simulink model "DC_AC"  (R2023a)
settings: Solver=VariableStepAuto  StartTime=0.0  StopTime=1.5  MaxStep=1e-4  RelTol=1e-3
libraries: spsMosfetLib x32, spsSeriesRLCBranchLib x29, simulink x25, spsCurrentMeasurementLib x11, spsVoltageMeasurementLib x9, spsDCVoltageSourceLib x8, spsIdealSwitchLib x5, spsDiodeLib x1, spspowerguiLib x1
(part 1 of 2)
settings Model: Creator=TangZhenYu  LastModifiedBy=TangZhenYu

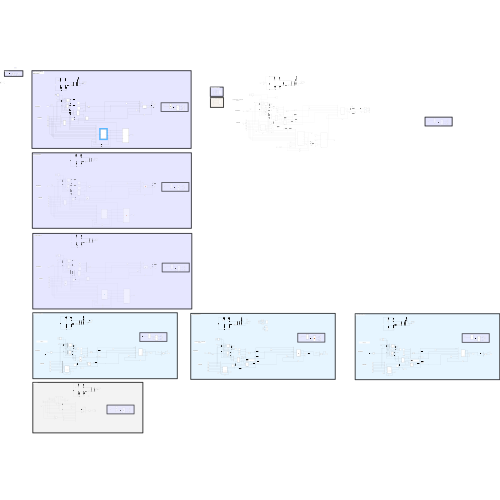
[thumbnail: Simulink's stored preview of the top-level diagram]
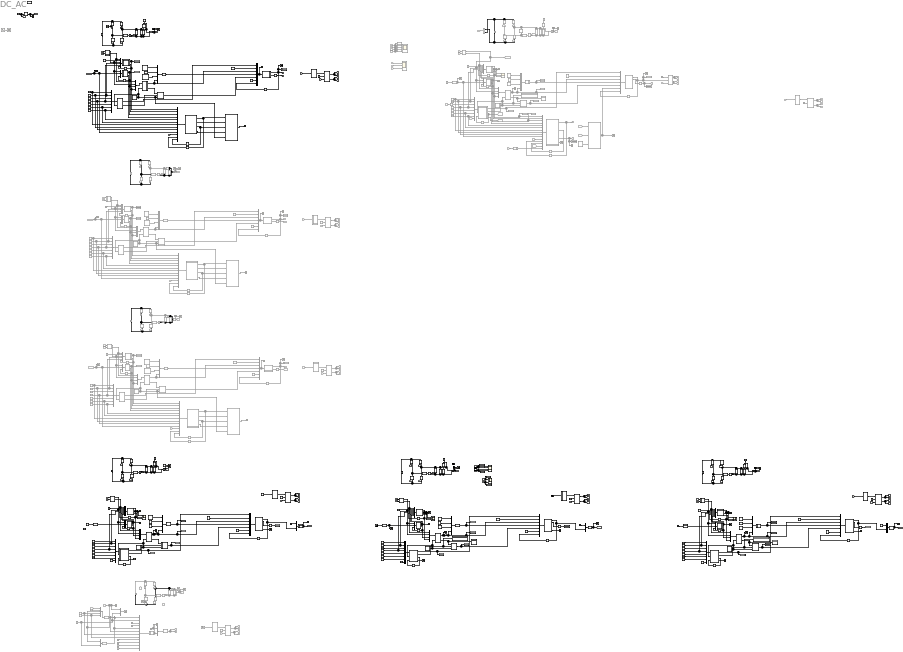
== system DC_AC ==
  note: 固定扰动下的电压跟踪效果
  note: 产生期望值
  note: 不同参数矩阵C下电压跟踪的状态
  note: C矩阵参数设置[1000,1]
  note: 最终驱动
  note: 电路参数
  note: 期望值修改
  note: 期望值修改
  note: 最终驱动
  note: 电路参数
  note: C矩阵参数设置[500,1],500的效果最好
  note: C矩阵参数设置[1500,1]
  note: 电路参数
  note: 最终驱动
  note: 期望值修改
  note: 注意代数环要延时一个机器周期的时间长度
  note: 期望值修改
  note: 电路参数
  note: 不考虑外部扰动的滑膜控制
  note: 最终驱动
  note: 传统的滑膜控制
  note: 最终驱动
  note: 注意代数环要延时一个机器周期的时间长度
  note: 电路参数
  note: 期望值修改
  note: 最终驱动
  note: 注意代数环要延时一个机器周期的时间长度
  note: 期望值修改
  note: 电路参数
  note: 不考虑外部扰动的滑膜控制
  note: 最终驱动
  note: 不考虑外部扰动的滑膜控制
  note: 期望值修改
  note: 最终驱动
  note: 注意代数环要延时一个机器周期的时间长度
  note: 电路参数
  (CΓ)'_Calculation : MATLAB Function  TreatAsAtomicUnit=on
  (CΓ)'_Calculation1 : MATLAB Function  Commented=on  TreatAsAtomicUnit=on
  (CΓ)'_Calculation2 : MATLAB Function  Commented=on  TreatAsAtomicUnit=on
  (CΓ)'_Calculation3 : MATLAB Function  TreatAsAtomicUnit=on
  (CΓ)'_Calculation4 : MATLAB Function  Commented=on  TreatAsAtomicUnit=on
  (CΓ)'_Calculation5 : MATLAB Function  TreatAsAtomicUnit=on
  (CΓ)'_Calculation6 : MATLAB Function  TreatAsAtomicUnit=on
  C : Constant  Commented=on  Value=1e-5
  C(电容值) : Constant  Value=1e-3
  C(电容值)1 : Constant  Commented=on  Value=1e-3
  C(电容值)2 : Constant  Commented=on  Value=1e-3
  C(电容值)3 : Constant  Value=0.0003
  C(电容值)4 : Constant  Commented=on  Value=0.0003
  C(电容值)5 : Constant  Value=0.0003
  C(电容值)6 : Constant  Value=0.0003
  C1 : Constant  Commented=on  Value=100
  C_Gamma_Inv1 : Display
  C_Gamma_Inv2 : Display
  C_Gamma_Inv3 : Display
  C_Gamma_Inv4 : Display  Commented=on
  Constant : Constant  Commented=on  Value=30
  Constant{1..5} (5 alike) : Constant  Commented=on  Value=0
  Current Measurement{1..3,6..7,12..13} (7 alike) : spsCurrentMeasurementLib/Current Measurement  Commented=on  PhasorSimulation=off  OutputType=Complex  PSBequivalent=0
  Current Measurement{4..5,8..9} (4 alike) : spsCurrentMeasurementLib/Current Measurement  PhasorSimulation=off  OutputType=Complex  PSBequivalent=0
  Cϕx1 : Display
  Cϕx2 : Display
  Cϕx3 : Display
  Cϕx4 : Display  Commented=on
  Cϕx_Calculation : MATLAB Function  TreatAsAtomicUnit=on
  Cϕx_Calculation1 : MATLAB Function  Commented=on  TreatAsAtomicUnit=on
  Cϕx_Calculation2 : MATLAB Function  Commented=on  TreatAsAtomicUnit=on
  Cϕx_Calculation3 : MATLAB Function  TreatAsAtomicUnit=on
  Cϕx_Calculation4 : MATLAB Function  Commented=on  TreatAsAtomicUnit=on
  Cϕx_Calculation5 : MATLAB Function  TreatAsAtomicUnit=on
  Cϕx_Calculation6 : MATLAB Function  TreatAsAtomicUnit=on
  DC Voltage Source1 : spsDCVoltageSourceLib/DC Voltage Source  Commented=on  Amplitude=80  Measurements=None
  DC Voltage Source2 : spsDCVoltageSourceLib/DC Voltage Source  Amplitude=80  Measurements=None
  DC Voltage Source3 : spsDCVoltageSourceLib/DC Voltage Source  Commented=on  Amplitude=80  Measurements=None
  DC Voltage Source4 : spsDCVoltageSourceLib/DC Voltage Source  Amplitude=80  Measurements=None
  DC Voltage Source5 : spsDCVoltageSourceLib/DC Voltage Source  Amplitude=85  Measurements=None
  DC Voltage Source6 : spsDCVoltageSourceLib/DC Voltage Source  Amplitude=85  Measurements=None
  DC Voltage Source7 : spsDCVoltageSourceLib/DC Voltage Source  Commented=on  Amplitude=50  Measurements=None
  DC Voltage Source9 : spsDCVoltageSourceLib/DC Voltage Source  Commented=on  Amplitude=80  Measurements=None
  Diode2 : spsDiodeLib/Diode  Commented=on  Ron=0.001  Lon=0  Vf=0.8  IC=0  UseSnubber=0  Rs=500  Cs=250e-9  Measurements=off
  Distrubance_Calculation : MATLAB Function  TreatAsAtomicUnit=on
  Distrubance_Calculation1 : MATLAB Function  TreatAsAtomicUnit=on
  Distrubance_Calculation2 : MATLAB Function  Commented=on  TreatAsAtomicUnit=on
  Distrubance_Calculation3 : MATLAB Function  Commented=on  TreatAsAtomicUnit=on
  Distrubance_Calculation4 : MATLAB Function  Commented=on  TreatAsAtomicUnit=on
  Distrubance_Calculation5 : MATLAB Function  Commented=on  TreatAsAtomicUnit=on
  Distrubance_Calculation6 : MATLAB Function  Commented=on  TreatAsAtomicUnit=on
  Distrubance_Calculation7 : MATLAB Function  Commented=on  TreatAsAtomicUnit=on
  E : Constant  Commented=on  Value=40
  E(实际的值){,3,5..6} (4 alike) : Constant  Value=70
  E(实际的值)1 : Constant  Commented=on  Value=80
  E(实际的值)2 : Constant  Commented=on  Value=80
  E(实际的值)4 : Constant  Commented=on  Value=70
  E_0(理论值){,3,5..6} (4 alike) : Constant  Value=70
  E_0(理论值)1 : Constant  Commented=on  Value=80
  E_0(理论值)2 : Constant  Commented=on  Value=80
  E_0(理论值)4 : Constant  Commented=on  Value=70
  From11 : From  Commented=on  GotoTag=Q1_2
  From14 : From  Commented=on  GotoTag=Q2_2
  From15 : From  Commented=on  GotoTag=u_k_2
  From16 : From  Commented=on  GotoTag=Q1_3
  From17 : From  Commented=on  GotoTag=Q2_3
  From18 : From  Commented=on  GotoTag=u_k_3
  From19 : From  Commented=on  GotoTag=Q3_3
  From20 : From  Commented=on  GotoTag=Q4_3
  From21 : From  Commented=on  GotoTag=u_k_1_3
  From22 : From  Commented=on  GotoTag=v_o_3
  From23 : From  Commented=on  GotoTag=i_l_3
  From24 : From  Commented=on  GotoTag=v_o
  From25 : From  Commented=on  GotoTag=v_o_2
  From26 : From  Commented=on  GotoTag=v_o_3
  From34 : From  Commented=on  GotoTag=i_l_5
  From35 : From  Commented=on  GotoTag=u_k_5
  From36 : From  Commented=on  GotoTag=v_o_5
  From38 : From  Commented=on  GotoTag=expect_value
  From39 : From  Commented=on  GotoTag=Q1_5
  From40 : From  Commented=on  GotoTag=Q2_5
  From41 : From  Commented=on  GotoTag=Q3_5
  From42 : From  Commented=on  GotoTag=Q4_5
  From43 : From  Commented=on  GotoTag=expect_value
  From{45..47,63,79} (5 alike) : From  Commented=on  GotoTag=expect
  From48 : From  Commented=on  GotoTag=v_o
  From49 : From  Commented=on  GotoTag=v_o_4
  From5 : From  Commented=on  GotoTag=Q3_2
  From50 : From  Commented=on  GotoTag=v_o_3
  From53 : From  Commented=on  GotoTag=i_l_6
  From54 : From  Commented=on  GotoTag=V_Output_6
  From55 : From  Commented=on  GotoTag=V_Input_6
  From56 : From  Commented=on  GotoTag=d1_6
  From57 : From  Commented=on  GotoTag=D_Disturb_k_1_6
  From58 : From  Commented=on  GotoTag=D_Disturb_k_2_6
  From59 : From  Commented=on  GotoTag=u_k_1_6
  From6 : From  Commented=on  GotoTag=Q4_2
  From64 : From  Commented=on  GotoTag=v_o_6
  From7 : From  Commented=on  GotoTag=u_k_1_2
  From73 : From  Commented=on  GotoTag=Q3_6
  From74 : From  Commented=on  GotoTag=Q4_6
  From75 : From  Commented=on  GotoTag=Q1_6
  From76 : From  Commented=on  GotoTag=Q2_6
  From8 : From  Commented=on  GotoTag=v_o_2
  From9 : From  Commented=on  GotoTag=i_l_2
  Goto : Goto  Commented=on  GotoTag=Q1_6
  Goto10 : Goto  Commented=on  GotoTag=i_l_2
  Goto11 : Goto  Commented=on  GotoTag=Q4_2
  Goto12 : Goto  Commented=on  GotoTag=Q1_2
  Goto15 : Goto  Commented=on  GotoTag=u_k_1_2
  Goto16 : Goto  Commented=on  GotoTag=u_k_2
  Goto17 : Goto  Commented=on  GotoTag=i_l_3
  Goto18 : Goto  Commented=on  GotoTag=Q4_3
  Goto19 : Goto  Commented=on  GotoTag=Q1_3
  Goto20 : Goto  Commented=on  GotoTag=u_k_1_3
  Goto21 : Goto  Commented=on  GotoTag=u_k_3
  Goto22 : Goto  Commented=on  GotoTag=v_o_3
  Goto23 : Goto  Commented=on  GotoTag=Q2_3
  Goto24 : Goto  Commented=on  GotoTag=Q3_3
  Goto3 : Goto  Commented=on  GotoTag=v_o_2
  Goto33 : Goto  Commented=on  GotoTag=Q4_5
  Goto34 : Goto  Commented=on  GotoTag=Q1_5
  Goto35 : Goto  Commented=on  GotoTag=i_l_5
  Goto36 : Goto  Commented=on  GotoTag=v_o_5
  Goto37 : Goto  Commented=on  GotoTag=Q2_5
  Goto38 : Goto  Commented=on  GotoTag=Q3_5
  Goto40 : Goto  Commented=on  GotoTag=Q4_5
  Goto41 : Goto  Commented=on  GotoTag=Q1_5
  Goto42 : Goto  Commented=on  GotoTag=u_k_1_6
  Goto44 : Goto  Commented=on  GotoTag=V_Output_6
  Goto45 : Goto  Commented=on  GotoTag=R_6
  Goto46 : Goto  Commented=on  GotoTag=V_Input_6
  Goto47 : Goto  Commented=on  GotoTag=d1_6
  Goto48 : Goto  Commented=on  GotoTag=D_Disturb_k_1_6
  Goto49 : Goto  Commented=on  GotoTag=D_Disturb_k_2_6
  Goto5 : Goto  Commented=on  GotoTag=Q2_2
  Goto50 : Goto  Commented=on  GotoTag=v_o_6
  Goto51 : Goto  Commented=on  GotoTag=i_l_6
  Goto52 : Goto  Commented=on  GotoTag=Q4_6
  Goto57 : Goto  Commented=on  GotoTag=Q2_6
  Goto58 : Goto  Commented=on  GotoTag=Q3_6
  Goto61 : Goto  Commented=on  GotoTag=Q4_6
  Goto62 : Goto  Commented=on  GotoTag=Q1_6
  Goto63 : Goto  Commented=on  GotoTag=Q2_6
  Goto64 : Goto  Commented=on  GotoTag=Q3_6
  Goto9 : Goto  Commented=on  GotoTag=Q3_2
  Ideal Switch{,1,3..4} (4 alike) : spsIdealSwitchLib/Ideal Switch  Ron=0.5  Lon=0  IC=0  Rs=1e5  Cs=inf  Measurements=off
  Ideal Switch2 : spsIdealSwitchLib/Ideal Switch  Commented=on  Ron=0.5  Lon=0  IC=0  Rs=1e5  Cs=inf  Measurements=off
  L : Constant  Commented=on  Value=0.05
  L(电感值){,3,5..6} (4 alike) : Constant  Value=0.00365
  L(电感值)1 : Constant  Commented=on  Value=5e-3
  L(电感值)2 : Constant  Commented=on  Value=5e-3
  L(电感值)4 : Constant  Commented=on  Value=0.00365
  MATLAB Function : MATLAB Function  TreatAsAtomicUnit=on
  MATLAB Function1 : MATLAB Function  TreatAsAtomicUnit=on
  MATLAB Function10 : MATLAB Function  Commented=on  TreatAsAtomicUnit=on
  MATLAB Function11 : MATLAB Function  Commented=on  TreatAsAtomicUnit=on
  MATLAB Function12 : MATLAB Function  TreatAsAtomicUnit=on
  MATLAB Function13 : MATLAB Function  TreatAsAtomicUnit=on
  MATLAB Function14 : MATLAB Function  TreatAsAtomicUnit=on
  MATLAB Function15 : MATLAB Function  TreatAsAtomicUnit=on
  MATLAB Function16 : MATLAB Function  TreatAsAtomicUnit=on
  MATLAB Function17 : MATLAB Function  TreatAsAtomicUnit=on
  MATLAB Function18 : MATLAB Function  Commented=on  TreatAsAtomicUnit=on
  MATLAB Function19 : MATLAB Function  Commented=on  TreatAsAtomicUnit=on
  MATLAB Function2 : MATLAB Function  Commented=on  TreatAsAtomicUnit=on
  MATLAB Function20 : MATLAB Function  TreatAsAtomicUnit=on
  MATLAB Function21 : MATLAB Function  Commented=on  TreatAsAtomicUnit=on
  MATLAB Function22 : MATLAB Function  TreatAsAtomicUnit=on
  MATLAB Function23 : MATLAB Function  TreatAsAtomicUnit=on
  MATLAB Function24 : MATLAB Function  TreatAsAtomicUnit=on
  MATLAB Function25 : MATLAB Function  Commented=on  TreatAsAtomicUnit=on
  MATLAB Function26 : MATLAB Function  Commented=on  TreatAsAtomicUnit=on
  MATLAB Function27 : MATLAB Function  Commented=on  TreatAsAtomicUnit=on
  MATLAB Function28 : MATLAB Function  Commented=on  TreatAsAtomicUnit=on
  MATLAB Function29 : MATLAB Function  TreatAsAtomicUnit=on
  MATLAB Function3 : MATLAB Function  Commented=on  TreatAsAtomicUnit=on
  MATLAB Function30 : MATLAB Function  TreatAsAtomicUnit=on
  MATLAB Function31 : MATLAB Function  TreatAsAtomicUnit=on
  MATLAB Function32 : MATLAB Function  TreatAsAtomicUnit=on
  MATLAB Function33 : MATLAB Function  TreatAsAtomicUnit=on
  MATLAB Function4 : MATLAB Function  TreatAsAtomicUnit=on
  MATLAB Function5 : MATLAB Function  TreatAsAtomicUnit=on
  MATLAB Function6 : MATLAB Function  Commented=on  TreatAsAtomicUnit=on
  MATLAB Function7 : MATLAB Function  Commented=on  TreatAsAtomicUnit=on
  MATLAB Function8 : MATLAB Function  Commented=on  TreatAsAtomicUnit=on
  MATLAB Function9 : MATLAB Function  Commented=on  TreatAsAtomicUnit=on
  Mosfet{1,6..12,22..25,27..30} (16 alike) : spsMosfetLib/Mosfet  Commented=on  Ron=0.1  Lon=0  Rd=0.01  Vfd=0  IC=0  Rs=1e5  Cs=inf  Measurements=off
  Mosfet{2..5,13..21,26,31..32} (16 alike) : spsMosfetLib/Mosfet  Ron=0.1  Lon=0  Rd=0.01  Vfd=0  IC=0  Rs=1e5  Cs=inf  Measurements=off
  Mux : Mux  Inputs=7
  Mux{1,5,23,27,42,46,49,53} (8 alike) : Mux
  Mux10 : Mux  Commented=on  Inputs=[1 1 1]
  Mux11 : Mux  Commented=on  Inputs=[1 1 1 1 1 1 1 1 1 1 1 1 1]
  Mux{8,12,16,19,34,38} (6 alike) : Mux  Commented=on
  Mux13 : Mux  Commented=on  Inputs=[1 1 1 1 1 1 1]
  Mux14 : Mux  Commented=on  Inputs=[1 1 1]
  Mux15 : Mux  Commented=on  Inputs=[1 1 1 1 1 1 1 1 1 1 1 1 1]
  Mux17 : Mux  Commented=on  Inputs=[1 1 1 1 1 1 1]
  Mux18 : Mux  Commented=on  Inputs=7
  Mux2 : Mux  Inputs=[1 1 1 1 1 1]
  Mux20 : Mux  Commented=on  Inputs=[1 1 1 1 1 1]
  Mux21 : Mux  Inputs=[1 1 1 1 1 1 1 1]
  Mux{3,22,41,48} (4 alike) : Mux  Inputs=[1 1 1]
  Mux{6,24,43,50} (4 alike) : Mux  Inputs=[1 1 1 1 1 1 1]
  Mux25 : Mux  Inputs=[1 1]
  Mux26 : Mux  Inputs=8
  Mux28 : Mux  Commented=on  Inputs=2
  Mux29 : Mux  Commented=on  Inputs=5
  Mux30 : Mux  Commented=on  Inputs=2
  Mux31 : Mux  Commented=on  Inputs=12
  Mux32 : Mux  Commented=on  Inputs=[1 1]
  Mux33 : Mux  Commented=on  Inputs=8
  Mux35 : Mux  Commented=on  Inputs=[1 1 1 1 1 1 1 1]
  Mux36 : Mux  Commented=on  Inputs=[1 1 1]
  Mux37 : Mux  Commented=on  Inputs=[1 1 1 1 1 1 1 1 1 1 1 1 1 1 1]
  Mux39 : Mux  Commented=on  Inputs=[1 1 1 1 1 1 1]
  Mux4 : Mux  Inputs=[1 1 1 1 1 1 1 1 1 1 1 1 1]
  Mux40 : Mux  Inputs=[1 1 1 1 1 1 1 1]
  Mux44 : Mux  Inputs=[1 1]
  Mux45 : Mux  Inputs=8
  Mux47 : Mux  Inputs=[1 1 1 1 1 1 1 1]
  Mux51 : Mux  Inputs=[1 1]
  Mux52 : Mux  Inputs=8
  Mux7 : Mux  Commented=on  Inputs=7
  Mux9 : Mux  Commented=on  Inputs=[1 1 1 1 1 1]
  Phi2 : Display  Commented=on
  Phi3 : Display
  Phi4 : Display
  R(实际值)1 : From  Commented=on  GotoTag=R_6
  R(实际的值) : Constant  Value=50
  R(实际的值)1 : Constant  Commented=on  Value=50
  R(实际的值)2 : Constant  Commented=on  Value=50
  R_0 : Constant  Commented=on  Value=60
  R_0(实际值)1 : Constant  Value=50
  R_0(实际值)2 : Constant  Commented=on  Value=50
  R_0(实际值)3 : Constant  Value=50
  R_0(实际值)4 : Constant  Value=50
  R_0(理论值) : Constant  Value=42
  R_0(理论值)1 : Constant  Commented=on  Value=50
  R_0(理论值)2 : Constant  Commented=on  Value=50
  R_0(理论值)3 : Constant  Value=50
  R_0(理论值)4 : Constant  Commented=on  Value=50
  R_0(理论值)5 : Constant  Value=50
  R_0(理论值)6 : Constant  Value=50
  Real_R_Value1 : Display  Commented=on
  Repeating Sequence Stair{,2..3,8} (4 alike) : simulink/Sources/Repeating Sequence Stair  OutValues=[0 1].'  tsamp=0.05  OutMin=[]  OutMax=[]  OutDataTypeStr=double  OutputDataTypeScalingMode=double  OutDataType=fixdt(0,8)  ConRadixGroup=Best Precision: Vector-wise  OutScaling=2^-12
  Repeating Sequence Stair1 : simulink/Sources/Repeating Sequence Stair  OutValues=[-40 40].'  tsamp=0.1  OutMin=[]  OutMax=[]  OutDataTypeStr=double  OutputDataTypeScalingMode=double  OutDataType=fixdt(0,8)  ConRadixGroup=Best Precision: Vector-wise  OutScaling=2^-12
  Repeating Sequence Stair10 : simulink/Sources/Repeating Sequence Stair  OutValues=[40.2 -40.2].'  tsamp=0.1  OutMin=[]  OutMax=[]  OutDataTypeStr=double  OutputDataTypeScalingMode=double  OutDataType=fixdt(0,8)  ConRadixGroup=Best Precision: Vector-wise  OutScaling=2^-12
  Repeating Sequence Stair11 : simulink/Sources/Repeating Sequence Stair  OutValues=[40.2 -40.2].'  tsamp=0.5  OutMin=[]  OutMax=[]  OutDataTypeStr=double  OutputDataTypeScalingMode=double  OutDataType=fixdt(0,8)  ConRadixGroup=Best Precision: Vector-wise  OutScaling=2^-12
  Repeating Sequence Stair4 : simulink/Sources/Repeating Sequence Stair  Commented=on  OutValues=[0 1].'  tsamp=0.05  OutMin=[]  OutMax=[]  OutDataTypeStr=double  OutputDataTypeScalingMode=double  OutDataType=fixdt(0,8)  ConRadixGroup=Best Precision: Vector-wise  OutScaling=2^-12
  Repeating Sequence Stair5 : simulink/Sources/Repeating Sequence Stair  OutValues=[40.2 -40.2].'  tsamp=0.5  OutMin=[]  OutMax=[]  OutDataTypeStr=double  OutputDataTypeScalingMode=double  OutDataType=fixdt(0,8)  ConRadixGroup=Best Precision: Vector-wise  OutScaling=2^-12
  Repeating Sequence Stair6 : simulink/Sources/Repeating Sequence Stair  OutValues=[40.2 -40.2].'  tsamp=0.5  OutMin=[]  OutMax=[]  OutDataTypeStr=double  OutputDataTypeScalingMode=double  OutDataType=fixdt(0,8)  ConRadixGroup=Best Precision: Vector-wise  OutScaling=2^-12
  Repeating Sequence Stair7 : simulink/Sources/Repeating Sequence Stair  Commented=on  OutValues=[40 -40].'  tsamp=0.1  OutMin=[]  OutMax=[]  OutDataTypeStr=double  OutputDataTypeScalingMode=double  OutDataType=fixdt(0,8)  ConRadixGroup=Best Precision: Vector-wise  OutScaling=2^-12
  Repeating Sequence Stair9 : simulink/Sources/Repeating Sequence Stair  OutValues=[-42 42].'  tsamp=0.1  OutMin=[]  OutMax=[]  OutDataTypeStr=double  OutputDataTypeScalingMode=double  OutDataType=fixdt(0,8)  ConRadixGroup=Best Precision: Vector-wise  OutScaling=2^-12
  Repeating Sequence1 : simulink/Sources/Repeating Sequence  Commented=on  rep_seq_t=[0 0.5/1000 1/1000]  rep_seq_y=[0 1 0]
  Repeating Sequence{2,5,10,12} (4 alike) : simulink/Sources/Repeating Sequence  rep_seq_t=[0 0.5/1000 1/1000]  rep_seq_y=[0 1 0]
  Repeating Sequence11 : simulink/Sources/Repeating Sequence  Commented=on  rep_seq_t=[0 0.5/1000 1/1000]  rep_seq_y=[0 1 0]
  Repeating Sequence13 : simulink/Sources/Repeating Sequence  rep_seq_t=[0 5e-4 10e-4]  rep_seq_y=[0 1.5 0]
  Repeating Sequence3 : simulink/Sources/Repeating Sequence  Commented=on  rep_seq_t=[0 0.5/1000 1/1000]  rep_seq_y=[0 1 0]
  Repeating Sequence4 : simulink/Sources/Repeating Sequence  rep_seq_t=[0 5e-4 10e-4]  rep_seq_y=[0 1.5 0]
  Repeating Sequence6 : simulink/Sources/Repeating Sequence  Commented=on  rep_seq_t=[0 5e-4 10e-4]  rep_seq_y=[0 1 0]
  Repeating Sequence7 : simulink/Sources/Repeating Sequence  Commented=on  rep_seq_t=[0 0.5/1000 1/1000]  rep_seq_y=[0 15 0]
  Repeating Sequence8 : simulink/Sources/Repeating Sequence  Commented=on  rep_seq_t=[0 5e-4 10e-4]  rep_seq_y=[0 1.5 0]
  Repeating Sequence9 : simulink/Sources/Repeating Sequence  rep_seq_t=[0 5e-4 10e-4]  rep_seq_y=[0 1.5 0]
  Scope{,17..18,50,59} (5 alike) : Scope  NumInputPorts=2
  Scope{1,10,30..31,38} (5 alike) : Scope  Commented=on  NumInputPorts=2
  Scope{6..9,11..14,16,21..22,33..34,39,41..44,49,61} (20 alike) : Scope  Commented=on
  Scope15 : Scope  Commented=on  NumInputPorts=4
  Scope{2..5,19,23..29,37,40,45..47,51,53..58,60} (25 alike) : Scope
  Scope20 : Scope  NumInputPorts=3
  Scope32 : Scope  Commented=on  NumInputPorts=3
  Scope35 : Scope  Commented=on  NumInputPorts=3
  Scope36 : Scope  NumInputPorts=3
  Scope48 : Scope  NumInputPorts=4
  Scope52 : Scope  NumInputPorts=3
  Series RLC Branch1 : spsSeriesRLCBranchLib/Series RLC Branch  Commented=on  LConnTagsString=__new0  RConnTagsString=__new0  BranchType=L  Resistance=1  Inductance=5e-3  SetiL0=off  InitialCurrent=0  Capacitance=1e-6  Setx0=off  InitialVoltage=0  Measurements=None
  Series RLC Branch10 : spsSeriesRLCBranchLib/Series RLC Branch  LConnTagsString=__new0  RConnTagsString=__new0  BranchType=R  Resistance=42  Inductance=1e-3  SetiL0=off  InitialCurrent=0  Capacitance=1e-6  Setx0=off  InitialVoltage=0  Measurements=None
  Series RLC Branch{9,11,15,18,26,29} (6 alike) : spsSeriesRLCBranchLib/Series RLC Branch  LConnTagsString=__new0  RConnTagsString=__new0  BranchType=R  Resistance=50  Inductance=1e-3  SetiL0=off  InitialCurrent=0  Capacitance=1e-6  Setx0=off  InitialVoltage=0  Measurements=None
  Series RLC Branch12 : spsSeriesRLCBranchLib/Series RLC Branch  LConnTagsString=__new0  RConnTagsString=__new0  BranchType=L  Resistance=1  Inductance=0.00365  SetiL0=off  InitialCurrent=0  Capacitance=1e-6  Setx0=off  InitialVoltage=0  Measurements=None
  Series RLC Branch13 : spsSeriesRLCBranchLib/Series RLC Branch  LConnTagsString=__new0  RConnTagsString=__new0  BranchType=C  Resistance=1  Inductance=1e-3  SetiL0=off  InitialCurrent=0  Capacitance=0.0003  Setx0=off  InitialVoltage=0  Measurements=None
  Series RLC Branch14 : spsSeriesRLCBranchLib/Series RLC Branch  LConnTagsString=__new0  RConnTagsString=__new0  BranchType=R  Resistance=42  Inductance=1e-3  SetiL0=off  InitialCurrent=0  Capacitance=1e-6  Setx0=off  InitialVoltage=0  Measurements=None
  Series RLC Branch16 : spsSeriesRLCBranchLib/Series RLC Branch  LConnTagsString=__new0  RConnTagsString=__new0  BranchType=L  Resistance=1  Inductance=5e-3  SetiL0=off  InitialCurrent=0  Capacitance=1e-6  Setx0=off  InitialVoltage=0  Measurements=None
  Series RLC Branch17 : spsSeriesRLCBranchLib/Series RLC Branch  LConnTagsString=__new0  RConnTagsString=__new0  BranchType=C  Resistance=1  Inductance=1e-3  SetiL0=off  InitialCurrent=0  Capacitance=1e-4  Setx0=off  InitialVoltage=0  Measurements=None
  Series RLC Branch19 : spsSeriesRLCBranchLib/Series RLC Branch  Commented=on  LConnTagsString=__new0  RConnTagsString=__new0  BranchType=R  Resistance=42  Inductance=1e-3  SetiL0=off  InitialCurrent=0  Capacitance=1e-6  Setx0=off  InitialVoltage=0  Measurements=None
  Series RLC Branch2 : spsSeriesRLCBranchLib/Series RLC Branch  Commented=on  LConnTagsString=__new0  RConnTagsString=__new0  BranchType=C  Resistance=1  Inductance=1e-3  SetiL0=off  InitialCurrent=0  Capacitance=1e-5  Setx0=off  InitialVoltage=0  Measurements=None
  Series RLC Branch20 : spsSeriesRLCBranchLib/Series RLC Branch  Commented=on  LConnTagsString=__new0  RConnTagsString=__new0  BranchType=L  Resistance=1  Inductance=0.05  SetiL0=off  InitialCurrent=0  Capacitance=1e-6  Setx0=off  InitialVoltage=0  Measurements=None
  Series RLC Branch21 : spsSeriesRLCBranchLib/Series RLC Branch  Commented=on  LConnTagsString=__new0  RConnTagsString=__new0  BranchType=C  Resistance=1  Inductance=1e-3  SetiL0=off  InitialCurrent=0  Capacitance=1e-5  Setx0=off  InitialVoltage=0  Measurements=None
  Series RLC Branch22 : spsSeriesRLCBranchLib/Series RLC Branch  Commented=on  LConnTagsString=__new0  RConnTagsString=__new0  BranchType=R  Resistance=50  Inductance=1e-3  SetiL0=off  InitialCurrent=0  Capacitance=1e-6  Setx0=off  InitialVoltage=0  Measurements=None
  Series RLC Branch23 : spsSeriesRLCBranchLib/Series RLC Branch  Commented=on  LConnTagsString=__new0  RConnTagsString=__new0  BranchType=L  Resistance=1  Inductance=0.00365  SetiL0=off  InitialCurrent=0  Capacitance=1e-6  Setx0=off  InitialVoltage=0  Measurements=None
  Series RLC Branch24 : spsSeriesRLCBranchLib/Series RLC Branch  Commented=on  LConnTagsString=__new0  RConnTagsString=__new0  BranchType=C  Resistance=1  Inductance=1e-3  SetiL0=off  InitialCurrent=0  Capacitance=0.0003  Setx0=off  InitialVoltage=0  Measurements=None
  Series RLC Branch25 : spsSeriesRLCBranchLib/Series RLC Branch  Commented=on  LConnTagsString=__new0  RConnTagsString=__new0  BranchType=R  Resistance=42  Inductance=1e-3  SetiL0=off  InitialCurrent=0  Capacitance=1e-6  Setx0=off  InitialVoltage=0  Measurements=None
  Series RLC Branch27 : spsSeriesRLCBranchLib/Series RLC Branch  LConnTagsString=__new0  RConnTagsString=__new0  BranchType=L  Resistance=1  Inductance=5e-3  SetiL0=off  InitialCurrent=0  Capacitance=1e-6  Setx0=off  InitialVoltage=0  Measurements=None
  Series RLC Branch28 : spsSeriesRLCBranchLib/Series RLC Branch  LConnTagsString=__new0  RConnTagsString=__new0  BranchType=C  Resistance=1  Inductance=1e-3  SetiL0=off  InitialCurrent=0  Capacitance=1e-4  Setx0=off  InitialVoltage=0  Measurements=None
  Series RLC Branch3 : spsSeriesRLCBranchLib/Series RLC Branch  Commented=on  LConnTagsString=__new0  RConnTagsString=__new0  BranchType=R  Resistance=50  Inductance=1e-3  SetiL0=off  InitialCurrent=0  Capacitance=1e-6  Setx0=off  InitialVoltage=0  Measurements=None
  Series RLC Branch4 : spsSeriesRLCBranchLib/Series RLC Branch  Commented=on  LConnTagsString=__new0  RConnTagsString=__new0  BranchType=L  Resistance=1  Inductance=5e-3  SetiL0=off  InitialCurrent=0  Capacitance=1e-6  Setx0=off  InitialVoltage=0  Measurements=None
  Series RLC Branch5 : spsSeriesRLCBranchLib/Series RLC Branch  Commented=on  LConnTagsString=__new0  RConnTagsString=__new0  BranchType=C  Resistance=1  Inductance=1e-3  SetiL0=off  InitialCurrent=0  Capacitance=1e-5  Setx0=off  InitialVoltage=0  Measurements=None
  Series RLC Branch6 : spsSeriesRLCBranchLib/Series RLC Branch  Commented=on  LConnTagsString=__new0  RConnTagsString=__new0  BranchType=R  Resistance=50  Inductance=1e-3  SetiL0=off  InitialCurrent=0  Capacitance=1e-6  Setx0=off  InitialVoltage=0  Measurements=None
  Series RLC Branch7 : spsSeriesRLCBranchLib/Series RLC Branch  LConnTagsString=__new0  RConnTagsString=__new0  BranchType=L  Resistance=1  Inductance=0.001323  SetiL0=off  InitialCurrent=0  Capacitance=1e-6  Setx0=off  InitialVoltage=0  Measurements=None
  Series RLC Branch8 : spsSeriesRLCBranchLib/Series RLC Branch  LConnTagsString=__new0  RConnTagsString=__new0  BranchType=C  Resistance=1  Inductance=1e-3  SetiL0=off  InitialCurrent=0  Capacitance=0.0003  Setx0=off  InitialVoltage=0  Measurements=None
  Sine Wave1 : Sin  Commented=on  Amplitude=60  SampleTime=0
  Sine Wave{6,10..12} (4 alike) : Sin  Amplitude=60  Frequency=20  SampleTime=0
  Sine Wave2 : Sin  Commented=on  Amplitude=60  Frequency=20  SampleTime=0
  Sine Wave3 : Sin  Commented=on  Amplitude=60  Frequency=20  SampleTime=0
  Sine Wave4 : Sin  Commented=on  Amplitude=60  Frequency=20  SampleTime=0
  Sine Wave5 : Sin  Commented=on  Amplitude=60  SampleTime=0
  Sine Wave7 : Sin  Amplitude=60  SampleTime=0
  Sine Wave8 : Sin  Amplitude=60  SampleTime=0
  Sine Wave9 : Sin  Commented=on  Amplitude=60  SampleTime=0
  Sk1 : Display
  Sk2 : Display
  Sk3 : Display
  Sk4 : Display  Commented=on
  Sk_Calculation : MATLAB Function  TreatAsAtomicUnit=on
  Sk_Calculation1 : MATLAB Function  Commented=on  TreatAsAtomicUnit=on
  Sk_Calculation2 : MATLAB Function  Commented=on  TreatAsAtomicUnit=on
  Sk_Calculation3 : MATLAB Function  TreatAsAtomicUnit=on
  Sk_Calculation4 : MATLAB Function  Commented=on  TreatAsAtomicUnit=on
  Sk_Calculation5 : MATLAB Function  TreatAsAtomicUnit=on
  Sk_Calculation6 : MATLAB Function  TreatAsAtomicUnit=on
  Sum : Sum  Commented=on  Inputs=|++
  To Workspace : ToWorkspace  Commented=on  VariableName=C500  SampleTime=-1
  To Workspace1 : ToWorkspace  Commented=on  VariableName=C1000  SampleTime=-1
  To Workspace2 : ToWorkspace  Commented=on  VariableName=C1500  SampleTime=-1
  To Workspace3 : ToWorkspace  Commented=on  VariableName=desert  SampleTime=-1
  To Workspace4 : ToWorkspace  VariableName=worst  SaveFormat=Timeseries  SampleTime=-1
  To Workspace5 : ToWorkspace  VariableName=medium  SaveFormat=Timeseries  SampleTime=-1
  To Workspace6 : ToWorkspace  VariableName=best  SaveFormat=Timeseries  SampleTime=-1
  To Workspace7 : ToWorkspace  VariableName=sbest  SaveFormat=Timeseries  SampleTime=-1
  To Workspace8 : ToWorkspace  VariableName=sworst  SaveFormat=Timeseries  SampleTime=-1
  Transport Delay1 : TransportDelay  DelayTime=0.0002
  Transport Delay{10..11,13..14} (4 alike) : TransportDelay  Commented=on  DelayTime=0.0003
  Transport Delay{8,12,15,17} (4 alike) : TransportDelay  Commented=on  DelayTime=0.0001
  Transport Delay{7,9,16,18} (4 alike) : TransportDelay  Commented=on  DelayTime=0.0002
  Transport Delay{19..23,31..40} (15 alike) : TransportDelay  DelayTime=1e-5
  Transport Delay2 : TransportDelay  DelayTime=0.0001
  Transport Delay{24..30} (7 alike) : TransportDelay  Commented=on  DelayTime=1e-5
  Transport Delay3 : TransportDelay  DelayTime=0.0002
  Transport Delay4 : TransportDelay  DelayTime=0.0003
  Transport Delay5 : TransportDelay  DelayTime=0.0003
  Transport Delay6 : TransportDelay  DelayTime=0.0001
  Voltage Measurement{1..2,5,7..8} (5 alike) : spsVoltageMeasurementLib/Voltage Measurement  Commented=on  PhasorSimulation=off  OutputType=Complex  PSBequivalent=0
  Voltage Measurement{3..4,6,9} (4 alike) : spsVoltageMeasurementLib/Voltage Measurement  PhasorSimulation=off  OutputType=Complex  PSBequivalent=0
  Vr_derise_d{,3,5..6} (4 alike) : Constant  Value=0
  Vr_derise_d1 : Constant  Commented=on  Value=0
  Vr_derise_d2 : Constant  Commented=on  Value=0
  Vr_derise_d4 : Constant  Commented=on  Value=0
  X_matrix2 : Display  Commented=on
  X_matrix3 : Display
  X_matrix4 : Display
  alfa(是一个0~1的数) : Constant  Value=0.5
  alfa(是一个0~1的数)1 : Constant  Commented=on  Value=0.5
  alfa(是一个0~1的数)2 : Constant  Commented=on  Value=0.5
  alfa(是一个0~1的数)3 : Constant  Value=0.25
  alfa(是一个0~1的数)4 : Constant  Commented=on  Value=0.25
  alfa(是一个0~1的数)5 : Constant  Value=0.25
  alfa(是一个0~1的数)6 : Constant  Value=0.25
  c_Matrix : Constant  Value=[0 0 1000 1]
  c_Matrix1 : Constant  Commented=on  Value=[0 0 1000 1]
  c_Matrix2 : Constant  Commented=on  Value=[0 0 1500 1]
  c_Matrix3 : Constant  Value=[0 0 1000 1]
  c_Matrix4 : Constant  Commented=on  Value=[0 0 1000 1]
  c_Matrix5 : Constant  Value=[0 0 1000 1]
  c_Matrix6 : Constant  Value=[0 0 500 1]
  c_Matrix_new1 : Constant  Commented=on  Value=[0 0 250 1]
  e1 : Display
  e1_Calculation : MATLAB Function  TreatAsAtomicUnit=on
  e1_Calculation1 : MATLAB Function  Commented=on  TreatAsAtomicUnit=on
  e1_Calculation2 : MATLAB Function  Commented=on  TreatAsAtomicUnit=on
  e1_Calculation3 : MATLAB Function  TreatAsAtomicUnit=on
  e1_Calculation4 : MATLAB Function  Commented=on  TreatAsAtomicUnit=on
  e1_Calculation5 : MATLAB Function  Commented=on  TreatAsAtomicUnit=on
  e1_Calculation6 : MATLAB Function  TreatAsAtomicUnit=on
  e1_Calculation7 : MATLAB Function  TreatAsAtomicUnit=on
  e2 : Display
  e2_Calculation : MATLAB Function  TreatAsAtomicUnit=on
  e2_Calculation1 : MATLAB Function  Commented=on  TreatAsAtomicUnit=on
  e2_Calculation2 : MATLAB Function  Commented=on  TreatAsAtomicUnit=on
  e2_Calculation3 : MATLAB Function  TreatAsAtomicUnit=on
  e2_Calculation4 : MATLAB Function  Commented=on  TreatAsAtomicUnit=on
  e2_Calculation5 : MATLAB Function  Commented=on  TreatAsAtomicUnit=on
  e2_Calculation6 : MATLAB Function  TreatAsAtomicUnit=on
  e2_Calculation7 : MATLAB Function  TreatAsAtomicUnit=on
  e{3..8} (6 alike) : Display  Commented=on
  h : Constant  Commented=on  Value=5e-4
  h(运算周期) : Constant  Value=1e-5
  h(运算周期)1 : Constant  Commented=on  Value=1e-5
  h(运算周期)2 : Constant  Commented=on  Value=1e-5
  h(运算周期)3 : Constant  Value=5e-4
  h(运算周期)4 : Constant  Value=0
  h(运算周期)5 : Constant  Commented=on  Value=5e-4
  h(运算周期)6 : Constant  Value=5e-4
  h(运算周期)7 : Constant  Value=0
  h(运算周期)8 : Constant  Value=5e-4
  h(运算周期)9 : Constant  Value=0
  l(是一个大于零的数){,3,5..6} (4 alike) : Constant
  l(是一个大于零的数)1 : Constant  Commented=on  Value=100
  l(是一个大于零的数)2 : Constant  Commented=on  Value=100
  l(是一个大于零的数)4 : Constant  Commented=on
  powergui : spspowerguiLib/powergui  Priority=1  SimulationMode=Discrete  SampleTime=1e-05  frequency=60  Iterations=50  frequencyindice=0  Pbase=100e6  ErrMax=1e-4  UnitsV=kV  UnitsW=MW  buscounter=0  FunctionMessages=off  echomessages=off  EnableUseOfTLC=off  CurrentSourceSwitches=off  DisableSnubberDevices=off  DisableRonSwitches=off  DisableVfSwitches=off  DisplayEquations=off  AutomaticDiscreteSolvers=off  SolverType=Tustin/Backward Euler (TBE)  Interpol=off  ExternalGateDelay=off  methode=off  Ts=100  x0status=blocks  SPID=on  SwTol=0  HookPort=off  NonlinearTolerance=1e-4  nMaxIteration=100  ContinueOnMaxIteration=off  RestoreLinks=warning  ResistiveCurrentMeasurement=off  Frange=[0:2:500]  Ylog=off  Xlog=on  ShowGrid=off  save=off  variable=ZData  structure=0  ZoomFFT=off  StartTime=0.0  cycles=1  DisplayStyle=1  fundamental=60  FreqAxis=off  MaxFrequency=1000  frequencyindicesteady=1  RmsSteady=1  display=off
  u(k)_Calculation : MATLAB Function  TreatAsAtomicUnit=on
  u(k)_Calculation1 : MATLAB Function  Commented=on  TreatAsAtomicUnit=on
  u(k)_Calculation2 : MATLAB Function  Commented=on  TreatAsAtomicUnit=on
  u(k)_Calculation3 : MATLAB Function  Commented=on  TreatAsAtomicUnit=on
  u(k)_Calculation_1 : MATLAB Function  TreatAsAtomicUnit=on
  u(k)_Calculation_2 : MATLAB Function  TreatAsAtomicUnit=on
  u(k)_Calculation_3 : MATLAB Function  TreatAsAtomicUnit=on
  u_Calculation : MATLAB Function  Commented=on  TreatAsAtomicUnit=on
  γgama(是一个0~1的数){,3,5..6} (4 alike) : Constant  Value=0.14
  γgama(是一个0~1的数)1 : Constant  Commented=on  Value=0.5
  γgama(是一个0~1的数)2 : Constant  Commented=on  Value=0.5
  γgama(是一个0~1的数)4 : Constant  Commented=on  Value=0.14
  δ/ϕ1 : Display
  δ/ϕ2 : Display
  δ/ϕ3 : Display
  δ/ϕ4 : Display  Commented=on
  δ/ϕ_Calculation : MATLAB Function  TreatAsAtomicUnit=on
  δ/ϕ_Calculation1 : MATLAB Function  Commented=on  TreatAsAtomicUnit=on
  δ/ϕ_Calculation2 : MATLAB Function  Commented=on  TreatAsAtomicUnit=on
  δ/ϕ_Calculation3 : MATLAB Function  TreatAsAtomicUnit=on
  δ/ϕ_Calculation4 : MATLAB Function  Commented=on  TreatAsAtomicUnit=on
  δ/ϕ_Calculation5 : MATLAB Function  TreatAsAtomicUnit=on
  δ/ϕ_Calculation6 : MATLAB Function  TreatAsAtomicUnit=on
  δdelta(是一个大于最大扰动的值){,3,5..6} (4 alike) : Constant  Value=60
  δdelta(是一个大于最大扰动的值)1 : Constant  Commented=on  Value=5
  δdelta(是一个大于最大扰动的值)2 : Constant  Commented=on  Value=5
  δdelta(是一个大于最大扰动的值)4 : Constant  Commented=on  Value=60
  不考虑外部扰动 : Constant  Value=0
  不考虑外部扰动1 : Constant  Commented=on  Value=0
  不考虑外部扰动2 : Constant  Commented=on  Value=0
  不考虑扰动1 : Constant  Value=0
  不考虑扰动2 : Constant  Value=0
  不考虑扰动3 : Constant  Value=0
  输出信号{,4,6..7} (4 alike) : Display
  输出信号{1..3,5} (4 alike) : Display  Commented=on
  wires:
  [Q4] -> Mosfet4/1
  [Q1] -> Mosfet3/1
  Current Measurement5/1 -> [i_l]
  Voltage Measurement6/1 -> Scope/2, [v_o]
  Mux3/1 -> e1_Calculation/1(u)
  E_0(理论值)/1 -> Mux4/6, Mux/6  "u(6)_E_0"
  Distrubance_Calculation/4(D2_K_2) -> Distrubance_Calculation1/4(D2_K_2)
  Mux/1 -> (CΓ)'_Calculation/1(u)
  MATLAB Function4/2(i_l) -> Mux5/1, Mux2/1  "Fact_i"
  E(实际的值)/1 -> Mux/5
  Cϕx_Calculation/1(y) -> Mux6/5  "u(5)_Cϕx"
  R(实际的值)/1 -> Mux/3
  e2_Calculation/2(Last_e2) -> Mux4/2  "u(2)_e2(k-1)"
  Transport Delay3/1 -> Mux4/12  "u(12)_d1(k-1)"
  Distrubance_Calculation1/1(C_d_Value) -> Scope5/1  "C_d_Value"
  Mux6/1 -> Scope4/1, u(k)_Calculation/1(u)
  R_0(理论值)/1 -> Mux2/5, Mux/4, Mux4/9  "u(9)_R_0"
  不考虑外部扰动/1 -> Mux6/6  "u(2)_alfa"
  alfa(是一个0~1的数)/1 -> Mux6/2  "u(2)_alfa"
  l(是一个大于零的数)/1 -> Mux1/3  "l"
  Transport Delay1/1 -> Mux4/13  "u(13)_d2(k-1)"
  Mux2/1 -> e2_Calculation/1(u)
  (CΓ)'_Calculation/2(Phi) -> Cϕx_Calculation/2(Phi)  "Phi"
  Mux1/1 -> δ/ϕ_Calculation/1(u)
  γgama(是一个0~1的数)/1 -> Mux1/2  "γgama"
  C(电容值)/1 -> Mux4/8, Mux2/4, Mux/2  "u(8)_C"
  e2_Calculation/1(Fact_e2) -> e2/1, Transport Delay6/1, Mux5/4, Mux4/1  "u(1)_e2(k)"
  h(运算周期)/1 -> Mux4/5, Mux/7  "u(5)_h"
  MATLAB Function4/1(v_o) -> Mux5/2, Mux3/1, Mux2/3  "Fact_V"
  Distrubance_Calculation/1(D1_K_1) -> Distrubance_Calculation1/1(D1_K_1), Transport Delay3/1  "d1(k-1)"
  Distrubance_Calculation/3(D2_K_1) -> Transport Delay1/1, Distrubance_Calculation1/3(D2_K_1)  "d2(k-1)"
  e1_Calculation/2(Last_e1) -> Mux4/4  "u(4)_e1(k-1)"
  Sk_Calculation/2(x_Matrix) -> Cϕx_Calculation/1(x_Matrix)  "x_Matrix"
  Mux5/1 -> Sk_Calculation/1(u)
  Sk_Calculation/1(Sk_Value) -> Mux6/3, Mux1/4  "u(3)_Sk_ValueSk"
  c_Matrix/1 -> (CΓ)'_Calculation/2(c), Sk_Calculation/2(c), Distrubance_Calculation1/5(c), Cϕx_Calculation/3(c_Matrix)  "c"
  δ/ϕ_Calculation/1(y) -> Mux6/4  "u(4)_δ/ϕ"
  [u_k_1] -> Mux4/11  "u(11)_u(k-1)"
  Distrubance_Calculation/2(D1_K_2) -> Distrubance_Calculation1/2(D1_K_2)
  Mux4/1 -> Distrubance_Calculation/1(u)
  Transport Delay4/1 -> Mux6/7  "u(7)_u_k-1"
  Transport Delay6/1 -> Mux2/6
  (CΓ)'_Calculation/1(C_Gamma_Inv) -> Mux6/1  "u(1)_PhiC_Gamma_Inv"
  e1_Calculation/1(Fact_e1) -> e1/1, Transport Delay2/1, Mux5/3, Mux4/3  "u(3)_e1(k)"
  δdelta(是一个大于最大扰动的值)/1 -> Mux1/1  "δdelta"
  Transport Delay2/1 -> Mux3/3
  Vr_derise_d/1 -> Mux2/2  "Vr_derise_d"
  u(k)_Calculation/2(u_k_1) -> Transport Delay5/1
  Transport Delay5/1 -> [u_k_1]
  L(电感值)/1 -> Mux4/7, Mux/1  "u(7)_L"
  u(k)_Calculation/1(u_k) -> 输出信号/1, Scope3/1, [u_k], Transport Delay4/1
  [v_o] -> MATLAB Function4/1(u)  "Fact_V"
  [i_l] -> MATLAB Function4/2(data)  "Fact_i"
  [expect_value] -> Scope2/1, Mux4/10, Mux3/2
  Sine Wave7/1 -> Scope/1  "u(10)_Vr_derise"
  MATLAB Function1/1(flag) -> MATLAB Function/1(flag)
  [expect] -> MATLAB Function1/1(desert)
  Repeating Sequence2/1 -> MATLAB Function/2(compare_data)
  MATLAB Function/1(Q14) -> [Q1], [Q4]
  MATLAB Function/2(Q23) -> [Q2], [Q3]
  [Q3] -> Scope28/1, Mosfet2/1
  [Q2] -> Mosfet5/1
  [u_k] -> MATLAB Function/3(u)
  Vr_derise_d1/1 -> Mux9/2  "Vr_derise_d"
  From15/1 -> MATLAB Function2/3(u)
  From5/1 -> Mosfet1/1
  Distrubance_Calculation2/4(D2_K_2) -> Distrubance_Calculation3/4(D2_K_2)
  Mux9/1 -> e2_Calculation1/1(u)
  From14/1 -> Mosfet8/1
  Sine Wave5/1 -> Scope1/1  "u(10)_Vr_derise"
  MATLAB Function6/1(v_o) -> Mux12/2, Mux10/1, Mux9/3  "Fact_V"
  From46/1 -> MATLAB Function3/1(desert)
  Repeating Sequence1/1 -> MATLAB Function2/2(compare_data)
  u(k)_Calculation1/1(u_k) -> 输出信号1/1, Scope7/1, Goto16/1, Transport Delay10/1
  l(是一个大于零的数)1/1 -> Mux8/3  "l"
  Sk_Calculation1/2(x_Matrix) -> Cϕx_Calculation1/1(x_Matrix)  "x_Matrix"
  From8/1 -> MATLAB Function6/1(u)  "Fact_V"
  MATLAB Function2/1(Q14) -> Goto12/1, Goto11/1
  Distrubance_Calculation2/2(D1_K_2) -> Distrubance_Calculation3/2(D1_K_2)
  L(电感值)1/1 -> Mux11/7, Mux7/1  "u(7)_L"
  From38/1 -> Scope6/1, Mux11/10, Mux10/2
  Mux12/1 -> Sk_Calculation1/1(u)
  MATLAB Function3/1(flag) -> MATLAB Function2/1(flag)
  From9/1 -> MATLAB Function6/2(data)  "Fact_i"
  Transport Delay11/1 -> Goto15/1
  e1_Calculation1/1(Fact_e1) -> e3/1, Transport Delay8/1, Mux12/3, Mux11/3  "u(3)_e1(k)"
  Transport Delay8/1 -> Mux10/3
  R(实际的值)1/1 -> Mux7/3
  Transport Delay10/1 -> Mux13/7  "u(7)_u_k-1"
  Sk_Calculation1/1(Sk_Value) -> Mux13/3, Mux8/4  "u(3)_Sk_ValueSk"
  From7/1 -> Mux11/11  "u(11)_u(k-1)"
  u(k)_Calculation1/2(u_k_1) -> Transport Delay11/1
  δdelta(是一个大于最大扰动的值)1/1 -> Mux8/1  "δdelta"
  e1_Calculation1/2(Last_e1) -> Mux11/4  "u(4)_e1(k-1)"
  Distrubance_Calculation2/1(D1_K_1) -> Distrubance_Calculation3/1(D1_K_1), Transport Delay9/1  "d1(k-1)"
  c_Matrix1/1 -> (CΓ)'_Calculation1/2(c), Sk_Calculation1/2(c), Distrubance_Calculation3/5(c), Cϕx_Calculation1/3(c_Matrix)  "c"
  e2_Calculation1/2(Last_e2) -> Mux11/2  "u(2)_e2(k-1)"
  MATLAB Function2/2(Q23) -> Goto5/1, Goto9/1
  δ/ϕ_Calculation1/1(y) -> Mux13/4  "u(4)_δ/ϕ"
  Distrubance_Calculation2/3(D2_K_1) -> Transport Delay7/1, Distrubance_Calculation3/3(D2_K_1)  "d2(k-1)"
  Mux11/1 -> Distrubance_Calculation2/1(u)
  Mux8/1 -> δ/ϕ_Calculation1/1(u)
  R_0(理论值)1/1 -> Mux9/5, Mux7/4, Mux11/9  "u(9)_R_0"
  alfa(是一个0~1的数)1/1 -> Mux13/2  "u(2)_alfa"
  C(电容值)1/1 -> Mux11/8, Mux9/4, Mux7/2  "u(8)_C"
  E(实际的值)1/1 -> Mux7/5
  γgama(是一个0~1的数)1/1 -> Mux8/2  "γgama"
  MATLAB Function6/2(i_l) -> Mux12/1, Mux9/1  "Fact_i"
  Mux13/1 -> Scope8/1, u(k)_Calculation1/1(u)
  E_0(理论值)1/1 -> Mux11/6, Mux7/6  "u(6)_E_0"
  不考虑外部扰动1/1 -> Mux13/6  "u(2)_alfa"
  Mux10/1 -> e1_Calculation1/1(u)
  Cϕx_Calculation1/1(y) -> Mux13/5  "u(5)_Cϕx"
  Voltage Measurement1/1 -> Scope1/2, Goto3/1
  h(运算周期)1/1 -> Mux11/5, Mux7/7  "u(5)_h"
  Current Measurement2/1 -> Goto10/1
  Distrubance_Calculation3/1(C_d_Value) -> Scope9/1  "C_d_Value"
  (CΓ)'_Calculation1/2(Phi) -> Cϕx_Calculation1/2(Phi)  "Phi"
  From11/1 -> Mosfet6/1
  Mux7/1 -> (CΓ)'_Calculation1/1(u)
  Transport Delay9/1 -> Mux11/12  "u(12)_d1(k-1)"
  From6/1 -> Mosfet7/1
  Transport Delay7/1 -> Mux11/13  "u(13)_d2(k-1)"
  (CΓ)'_Calculation1/1(C_Gamma_Inv) -> Mux13/1  "u(1)_PhiC_Gamma_Inv"
  e2_Calculation1/1(Fact_e2) -> e4/1, Transport Delay12/1, Mux12/4, Mux11/1  "u(1)_e2(k)"
  Transport Delay12/1 -> Mux9/6
  γgama(是一个0~1的数)2/1 -> Mux19/2  "γgama"
  MATLAB Function10/2(i_l) -> Mux16/1, Mux20/1  "Fact_i"
  alfa(是一个0~1的数)2/1 -> Mux17/2  "u(2)_alfa"
  C(电容值)2/1 -> Mux15/8, Mux20/4, Mux18/2  "u(8)_C"
  Mux19/1 -> δ/ϕ_Calculation2/1(u)
  Distrubance_Calculation4/3(D2_K_1) -> Transport Delay16/1, Distrubance_Calculation5/3(D2_K_1)  "d2(k-1)"
  MATLAB Function8/2(Q23) -> Goto23/1, Goto24/1
  δ/ϕ_Calculation2/1(y) -> Mux17/4  "u(4)_δ/ϕ"
  c_Matrix2/1 -> (CΓ)'_Calculation2/2(c), Sk_Calculation2/2(c), Distrubance_Calculation5/5(c), Cϕx_Calculation2/3(c_Matrix)  "c"
  e2_Calculation2/2(Last_e2) -> Mux15/2  "u(2)_e2(k-1)"
  (CΓ)'_Calculation2/1(C_Gamma_Inv) -> Mux17/1  "u(1)_PhiC_Gamma_Inv"
  Mux18/1 -> (CΓ)'_Calculation2/1(u)
  From16/1 -> Mosfet10/1
  h(运算周期)2/1 -> Mux15/5, Mux18/7  "u(5)_h"
  Current Measurement6/1 -> Goto17/1
  Voltage Measurement2/1 -> Scope10/2, Goto22/1
  Cϕx_Calculation2/1(y) -> Mux17/5  "u(5)_Cϕx"
  Mux14/1 -> e1_Calculation2/1(u)
  不考虑外部扰动2/1 -> Mux17/6  "u(2)_alfa"
  E_0(理论值)2/1 -> Mux15/6, Mux18/6  "u(6)_E_0"
  Sk_Calculation2/1(Sk_Value) -> Mux17/3, Mux19/4  "u(3)_Sk_ValueSk"
  Mux15/1 -> Distrubance_Calculation4/1(u)
  Distrubance_Calculation4/1(D1_K_1) -> Distrubance_Calculation5/1(D1_K_1), Transport Delay18/1  "d1(k-1)"
  Transport Delay13/1 -> Mux17/7  "u(7)_u_k-1"
  e2_Calculation2/1(Fact_e2) -> e6/1, Transport Delay15/1, Mux16/4, Mux15/1  "u(1)_e2(k)"
  Transport Delay15/1 -> Mux20/6
  u(k)_Calculation2/2(u_k_1) -> Transport Delay14/1
  δdelta(是一个大于最大扰动的值)2/1 -> Mux19/1  "δdelta"
  Transport Delay14/1 -> Goto20/1
  From43/1 -> Scope11/1, Mux15/10, Mux14/2
  MATLAB Function9/1(flag) -> MATLAB Function8/1(flag)
  From23/1 -> MATLAB Function10/2(data)  "Fact_i"
  Mux17/1 -> Scope13/1, u(k)_Calculation2/1(u)
  L(电感值)2/1 -> Mux15/7, Mux18/1  "u(7)_L"
  MATLAB Function8/1(Q14) -> Goto19/1, Goto18/1
  Distrubance_Calculation5/1(C_d_Value) -> Scope14/1  "C_d_Value"
  R_0(理论值)2/1 -> Mux20/5, Mux18/4, Mux15/9  "u(9)_R_0"
  Distrubance_Calculation4/2(D1_K_2) -> Distrubance_Calculation5/2(D1_K_2)
  Sk_Calculation2/2(x_Matrix) -> Cϕx_Calculation2/1(x_Matrix)  "x_Matrix"
  MATLAB Function10/1(v_o) -> Mux16/2, Mux14/1, Mux20/3  "Fact_V"
  Sine Wave9/1 -> Scope10/1  "u(10)_Vr_derise"
  e1_Calculation2/2(Last_e1) -> Mux15/4  "u(4)_e1(k-1)"
  From17/1 -> Mosfet12/1
  From19/1 -> Mosfet9/1
  Distrubance_Calculation4/4(D2_K_2) -> Distrubance_Calculation5/4(D2_K_2)
  Mux16/1 -> Sk_Calculation2/1(u)
  Vr_derise_d2/1 -> Mux20/2  "Vr_derise_d"
  From20/1 -> Mosfet11/1
  Repeating Sequence3/1 -> MATLAB Function8/2(compare_data)
  Transport Delay18/1 -> Mux15/12  "u(12)_d1(k-1)"
  Transport Delay16/1 -> Mux15/13  "u(13)_d2(k-1)"
  Mux20/1 -> e2_Calculation2/1(u)
  (CΓ)'_Calculation2/2(Phi) -> Cϕx_Calculation2/2(Phi)  "Phi"
  R(实际的值)2/1 -> Mux18/3
  E(实际的值)2/1 -> Mux18/5
  Transport Delay17/1 -> Mux14/3
  e1_Calculation2/1(Fact_e1) -> e5/1, Transport Delay17/1, Mux16/3, Mux15/3  "u(3)_e1(k)"
  From18/1 -> MATLAB Function8/3(u)
  l(是一个大于零的数)2/1 -> Mux19/3  "l"
  u(k)_Calculation2/1(u_k) -> 输出信号2/1, Scope12/1, Goto21/1, Transport Delay13/1
  From47/1 -> MATLAB Function9/1(desert)
  From21/1 -> Mux15/11  "u(11)_u(k-1)"
  From22/1 -> MATLAB Function10/1(u)  "Fact_V"
  From24/1 -> To Workspace/1, Scope15/1  "Fact_V"
  From25/1 -> To Workspace1/1, Scope15/2  "Fact_V"
  From26/1 -> To Workspace2/1, Scope15/3  "Fact_V"
  From45/1 -> To Workspace3/1, Scope15/4  "u(10)_Vr_derise"
  e2_Calculation3/4(Vo_RC) -> Scope20/2  "VO/RC"
  Mux22/1 -> e1_Calculation3/1(u)
  Mux23/1 -> Sk_Calculation3/1(u)
  Transport Delay20/1 -> 输出信号4/1
  δ/ϕ_Calculation3/1(y) -> Mux24/4, δ/ϕ2/1  "u(4)_δ/ϕ"
  Repeating Sequence4/1 -> Mux25/1
  Mux27/1 -> δ/ϕ_Calculation3/1(u)
  e2_Calculation3/1(Fact_e2) -> Scope20/3, Scope19/1, Mux23/4, Transport Delay21/1  "(IL/C)-VO/RC"
  e2_Calculation3/3(iL_C) -> Scope20/1  "IL/C"
  Vr_derise_d3/1 -> Mux21/2  "Vr_derise_d"
  Mux25/1 -> MATLAB Function12/1(u)
  Mux26/1 -> (CΓ)'_Calculation3/1(u)
  u(k)_Calculation_2/6(Disturbance) -> Scope29/1
  Mux21/1 -> e2_Calculation3/1(u)
  e1_Calculation3/1(Fact_e1) -> Mux21/7, Scope25/1, Mux23/3, Transport Delay23/1  "u(3)_e1(k)"
  u(k)_Calculation_2/2(u_k_1) -> Transport Delay20/1
  h(运算周期)4/1 -> Mux26/8  "u(5)_h"
  Transport Delay21/1 -> Mux21/6
  MATLAB Function17/1(y) -> Mux22/2  "u(10)_Vr_derise"
  Mux24/1 -> u(k)_Calculation_2/1(u)
  不考虑扰动1/1 -> Mux24/6  "u(2)_alfa"
  Sk_Calculation3/1(Sk_Value) -> Scope24/1, [Sk_1], Mux27/4, Sk2/1, Mux24/3  "conditional adpat SMC"
  Transport Delay19/1 -> Mux24/7  "u(7)_u_k-1"
  E_0(理论值)3/1 -> Mux26/6  "u(6)_E_0"
  R_0(实际值)1/1 -> Mux26/3  "u(9)_R_0"
  Sk_Calculation3/2(x_Matrix) -> Cϕx_Calculation3/1(x_Matrix)  "x_Matrix"
  e1_Calculation3/2(Last_e1) -> Mux21/8  "u(4)_e1(k-1)"
  alfa(是一个0~1的数)3/1 -> Mux24/2  "u(2)_alfa"
  Transport Delay23/1 -> Mux22/3
  (CΓ)'_Calculation3/4(D_Disturbance1_Matrix_k_2) -> Scope60/1
  C(电容值)3/1 -> Mux21/4, Mux26/2  "u(8)_C"
  MATLAB Function13/1(v_o) -> Mux22/1, Mux23/2, Mux21/3  "No_Consider_Disturbance"
  MATLAB Function12/1(Output) -> Scope26/1, [u_k_4]  "gate"
  u(k)_Calculation_2/1(u_k) -> Transport Delay19/1, Mux25/2  "u(k)"
  Cϕx_Calculation3/1(C_Phi_x) -> Cϕx2/1, Mux24/5  "u(5)_Cϕx"
  δdelta(是一个大于最大扰动的值)3/1 -> Mux27/1  "δdelta"
  Transport Delay22/1 -> (CΓ)'_Calculation3/3(D_k_1)
  (CΓ)'_Calculation3/2(Phi) -> Cϕx_Calculation3/2(Phi)  "Phi"
  γgama(是一个0~1的数)3/1 -> Mux27/2  "γgama"
  (CΓ)'_Calculation3/1(C_Gamma_Inv) -> C_Gamma_Inv2/1, Mux24/1  "u(1)_PhiC_Gamma_Inv"
  l(是一个大于零的数)3/1 -> Mux27/3  "l"
  E(实际的值)3/1 -> Mux26/5
  (CΓ)'_Calculation3/3(D_Disturbance1_Matrix_k_1) -> Transport Delay22/1
  R_0(理论值)3/1 -> Mux21/5, Mux26/4  "u(9)_R_0"
  L(电感值)3/1 -> Mux26/1  "u(7)_L"
  c_Matrix3/1 -> (CΓ)'_Calculation3/2(c), Sk_Calculation3/2(c), Cϕx_Calculation3/3(c_Matrix)  "c"
  h(运算周期)3/1 -> Mux26/7  "u(5)_h"
  Voltage Measurement3/1 -> Scope17/2, [v_o_4]
  Repeating Sequence Stair6/1 -> Scope17/1  "u(10)_Vr_derise"
  [Q3_4] -> Mosfet16/1
  [Q1_4] -> Mosfet13/1
  Current Measurement8/1 -> [i_l_4]
  [Q4_4] -> Mosfet14/1
  [Q2_4] -> Mosfet15/1
  [v_o_4] -> MATLAB Function13/1(u)  "Fact_V"
  [i_l_4] -> MATLAB Function13/2(data)  "Fact_i"
  MATLAB Function13/2(i_l) -> Mux23/1, Mux21/1  "Fact_i"
  [u_k_4] -> MATLAB Function14/3(u)
  Repeating Sequence5/1 -> MATLAB Function14/2(compare_data)
  MATLAB Function14/1(Q14) -> [Q1_4], [Q4_4]
  MATLAB Function14/2(Q23) -> [Q2_4], [Q3_4]
  Repeating Sequence Stair11/1 -> MATLAB Function15/1(desert)
  MATLAB Function15/1(flag) -> MATLAB Function14/1(flag)
  Mux28/1 -> Scope21/1
  Constant1/1 -> Mux29/2  "Vr_derise_d"
  Constant2/1 -> Mux31/4  "Vr_derise_dd"
  Mux30/1 -> e1_Calculation4/1(u)
  e2_Calculation4/1(y) -> Mux31/6, Sum/1  "e2"
  Mux31/1 -> u_Calculation/1(u)
  Mux29/1 -> e2_Calculation4/1(u)
  From36/1 -> Mux28/1, Scope16/1, Mux29/3, Mux30/1  "Conditional_SMC_Control"
  e1_Calculation4/1(y) -> Sum/2, Mux31/5  "e1"
  Constant/1 -> Mux30/2, Mux31/2, Mux28/2  "Vr_derise"
  Sum/1 -> Mux31/1  "s(k)"
  Constant3/1 -> Mux31/3  "Vr_derise_d"
  E/1 -> Mux31/10  "E"
  From34/1 -> Mux29/1  "fact_i"
  L/1 -> Mux31/9  "L"
  C1/1 -> Mux31/12  "C1"
  h/1 -> Mux31/11  "h"
  C/1 -> Mux31/8, Mux29/5  "C"
  u_Calculation/1(y) -> Scope31/2, Mux32/2
  R_0/1 -> Mux31/7, Mux29/4  "R_0"
  Constant5/1 -> Mosfet24/1
  Voltage Measurement7/1 -> Scope30/2, Goto36/1
  Constant4/1 -> Mosfet25/1
  Sine Wave2/1 -> Scope30/1  "u(10)_Vr_derise"
  From39/1 -> Scope33/1, Mosfet22/1
  Current Measurement13/1 -> Goto35/1
  From42/1 -> Mosfet23/1
  Repeating Sequence Stair5/1 -> MATLAB Function17/1(u)  "u(10)_Vr_derise"
  MATLAB Function19/1(flag) -> MATLAB Function18/1(flag)
  Sine Wave3/1 -> MATLAB Function19/1(desert)
  From35/1 -> MATLAB Function18/3(u)
  MATLAB Function18/2(Q23) -> Goto37/1, Goto38/1
  Repeating Sequence7/1 -> MATLAB Function18/2(compare_data)
  MATLAB Function18/1(Q14) -> Goto34/1, Goto33/1
  Repeating Sequence Stair1/1 -> [expect], MATLAB Function5/1(u)  "u(10)_Vr_derise"
  MATLAB Function5/1(y) -> Scope23/1, [expect_value]
  Repeating Sequence6/1 -> Scope31/1, Mux32/1
  Mux32/1 -> MATLAB Function7/1(u)
  MATLAB Function7/1(Output) -> Goto40/1, Goto41/1  "gate"
  From48/1 -> Scope32/1  "Fact_V"
  From49/1 -> Scope32/2  "Fact_V"
  From50/1 -> Scope32/3  "Fact_V"
  Repeating Sequence Stair/1 -> Ideal Switch/1
  Repeating Sequence Stair2/1 -> Ideal Switch1/1
  e2_Calculation5/4(Vo_RC) -> Scope35/2  "VO/RC"
  From56/1 -> Mux33/8  "u(14)_V_Output"
  E_0(理论值)4/1 -> Mux37/6, Mux33/6  "u(6)_E_0"
  Mux33/1 -> (CΓ)'_Calculation4/1(u)
  From57/1 -> Distrubance_Calculation7/1(D1_K_1)
  e1_Calculation5/1(Fact_e1) -> Mux35/7, Scope44/1, e7/1, Mux37/3, Mux38/3, Transport Delay24/1  "u(3)_e1(k)"
  Mux37/1 -> Distrubance_Calculation6/1(u)
  Transport Delay29/1 -> (CΓ)'_Calculation4/3(D_k_1)
  Mux39/1 -> u(k)_Calculation3/1(u)
  e2_Calculation5/1(Fact_e2) -> Scope35/3, Scope34/1, e8/1, Mux37/1, Mux38/4, Transport Delay28/1  "(IL/C)-VO/RC"
  l(是一个大于零的数)4/1 -> Mux34/3  "l"
  Mux34/1 -> δ/ϕ_Calculation4/1(u)
  δ/ϕ_Calculation4/1(y) -> Mux39/4, δ/ϕ4/1  "u(4)_δ/ϕ"
  Transport Delay26/1 -> Mux39/7  "u(7)_u_k-1"
  Mux38/1 -> Sk_Calculation4/1(u)
  MATLAB Function21/2(i_l) -> Mux38/1, Mux35/1  "Fact_i"
  Sk_Calculation4/1(Sk_Value) -> Scope43/1, Mux34/4, Sk4/1, Mux39/3  "improve"
  Repeating Sequence8/1 -> MATLAB Function11/1(compare)
  Mux36/1 -> e1_Calculation5/1(u)
  MATLAB Function21/1(v_o) -> Goto44/1, Mux36/1, Mux38/2, Mux35/3  "c=1000"
  Vr_derise_d4/1 -> Mux35/2  "Vr_derise_d"
  c_Matrix_new1/1 -> Distrubance_Calculation7/3(c)  "c"
  Transport Delay24/1 -> Mux36/3
  E(实际的值)4/1 -> Mux33/5
  Cϕx_Calculation4/1(C_Phi_x) -> Cϕx4/1, Mux39/5  "u(5)_Cϕx"
  Distrubance_Calculation7/1(C_d_Value) -> Mux39/6, Scope39/1  "u(6)_C_d_Value"
  (CΓ)'_Calculation4/1(C_Gamma_Inv) -> C_Gamma_Inv4/1, Mux39/1  "u(1)_PhiC_Gamma_Inv"
  Sk_Calculation4/2(x_Matrix) -> Cϕx_Calculation4/1(x_Matrix), X_matrix2/1  "x_Matrix"
  γgama(是一个0~1的数)4/1 -> Mux34/2  "γgama"
  h(运算周期)5/1 -> Mux37/5, Mux33/7  "u(5)_h"
  alfa(是一个0~1的数)4/1 -> Mux39/2  "u(2)_alfa"
  δdelta(是一个大于最大扰动的值)4/1 -> Mux34/1  "δdelta"
  From58/1 -> Distrubance_Calculation7/2(D1_K_2)
  Distrubance_Calculation6/6(Real_E_Value) -> Scope42/1
  C(电容值)4/1 -> Mux37/8, Mux35/4, Mux33/2  "u(8)_C"
  Distrubance_Calculation6/5(Real_R_Value) -> Scope41/1, Real_R_Value1/1, Goto45/1
  R_0(理论值)4/1 -> Mux37/9, Mux35/5, Mux33/4  "u(9)_R_0"
  Transport Delay28/1 -> Mux35/6
  Transport Delay30/1 -> Mux37/13  "u(13)_d2(k-1)"
  Transport Delay27/1 -> 输出信号5/1, Goto42/1
  Mux35/1 -> e2_Calculation5/1(u)
  MATLAB Function11/1(Q14) -> Goto/1, Goto52/1  "gate"
  Transport Delay25/1 -> Mux37/12  "u(12)_d1(k-1)"
  From59/1 -> Mux37/11  "u(11)_u(k-1)"
  u(k)_Calculation3/2(u_k_1) -> Transport Delay27/1
  Distrubance_Calculation6/3(D2_K_1) -> Transport Delay30/1
  e1_Calculation5/2(Last_e1) -> Mux35/8, Mux37/4  "u(4)_e1(k-1)"
  From54/1 -> Mux37/14  "u(14)_V_Output"
  u(k)_Calculation3/1(u_k) -> Transport Delay26/1, MATLAB Function11/2(u_k), 输出信号3/1, Scope22/1  "u(k)"
  R(实际值)1/1 -> Mux33/3
  (CΓ)'_Calculation4/2(Phi) -> Cϕx_Calculation4/2(Phi), Phi2/1  "Phi"
  MATLAB Function27/1(y) -> Scope49/1, Mux37/10, Mux36/2  "u(10)_Vr_derise"
  (CΓ)'_Calculation4/3(D_Disturbance1_Matrix_k_1) -> Transport Delay29/1, Goto48/1
  e2_Calculation5/2(Last_e2) -> Mux37/2  "u(2)_e2(k-1)"
  L(电感值)4/1 -> Mux37/7, Mux33/1  "u(7)_L"
  e2_Calculation5/3(iL_C) -> Scope35/1  "IL/C"
  Distrubance_Calculation6/1(D1_K_1) -> Goto47/1, Transport Delay25/1  "d1(k-1)"
  c_Matrix4/1 -> (CΓ)'_Calculation4/2(c), Sk_Calculation4/2(c), Cϕx_Calculation4/3(c_Matrix)  "c"
  (CΓ)'_Calculation4/4(D_Disturbance1_Matrix_k_2) -> Goto49/1
  Sine Wave1/1 -> Scope38/1  "u(10)_Vr_derise"
  Repeating Sequence Stair4/1 -> Ideal Switch2/1
  Voltage Measurement8/1 -> Scope38/2, Goto50/1
  Current Measurement7/1 -> Goto51/1
  From75/1 -> Mosfet28/1
  From74/1 -> Mosfet29/1
  Voltage Measurement5/1 -> Goto46/1  "Fact_V"
  From53/1 -> MATLAB Function21/2(data)  "Fact_i"
  From64/1 -> MATLAB Function21/1(u)  "c=1000"
  MATLAB Function11/2(Q23) -> Goto57/1, Goto58/1
  From63/1 -> MATLAB Function11/3(expect)
  From73/1 -> Mosfet27/1
  From76/1 -> Mosfet30/1
  MATLAB Function16/1(Output) -> Scope45/1, [u_k_7]  "gate"
  Transport Delay35/1 -> Mux41/3
  Repeating Sequence10/1 -> MATLAB Function22/2(compare_data)
  (CΓ)'_Calculation5/3(D_Disturbance1_Matrix_k_1) -> Transport Delay34/1
  Mux46/1 -> δ/ϕ_Calculation5/1(u)
  MATLAB Function22/1(Q14) -> [Q1_7], [Q4_7]
  MATLAB Function23/1(flag) -> MATLAB Function22/1(flag)
  [i_l_7] -> MATLAB Function20/2(data)  "Fact_i"
  [v_o_7] -> MATLAB Function20/1(u)  "Fact_V"
  Mux45/1 -> (CΓ)'_Calculation5/1(u)
  [u_k_7] -> MATLAB Function22/3(u)
  c_Matrix5/1 -> (CΓ)'_Calculation5/2(c), Sk_Calculation5/2(c), Cϕx_Calculation5/3(c_Matrix)  "c"
  MATLAB Function20/2(i_l) -> Mux42/1, Mux40/1  "Fact_i"
  [Q3_7] -> Mosfet20/1
  Current Measurement4/1 -> [i_l_7]
  [Q1_7] -> Mosfet17/1
  Sine Wave12/1 -> MATLAB Function23/1(desert)
  Mux44/1 -> MATLAB Function16/1(u)
  l(是一个大于零的数)5/1 -> Mux46/3  "l"
  E(实际的值)5/1 -> Mux45/5
  R_0(理论值)5/1 -> Mux40/5, Mux45/4  "u(9)_R_0"
  (CΓ)'_Calculation5/2(Phi) -> Cϕx_Calculation5/2(Phi), Phi3/1  "Phi"
  u(k)_Calculation_1/1(u_k) -> Transport Delay31/1, Mux44/2  "u(k)"
  alfa(是一个0~1的数)5/1 -> Mux43/2  "u(2)_alfa"
  γgama(是一个0~1的数)5/1 -> Mux46/2  "γgama"
  R_0(实际值)3/1 -> Mux45/3  "u(9)_R_0"
  Cϕx_Calculation5/1(C_Phi_x) -> Cϕx1/1, Mux43/5  "u(5)_Cϕx"
  e1_Calculation6/2(Last_e1) -> Mux40/8  "u(4)_e1(k-1)"
  e2_Calculation6/1(Fact_e2) -> Scope36/3, Scope27/1, Mux42/4, Transport Delay33/1  "(IL/C)-VO/RC"
  Sk_Calculation5/1(Sk_Value) -> Scope37/1, [Sk_2], Mux46/4, Sk1/1, Mux43/3  "conditional adpat SMC"
  u(k)_Calculation_1/6(Disturbance) -> Scope46/1
  不考虑扰动2/1 -> Mux43/6  "u(2)_alfa"
  e2_Calculation6/3(iL_C) -> Scope36/1  "IL/C"
  Mux41/1 -> e1_Calculation6/1(u)
  MATLAB Function24/1(y) -> Scope58/1, Mux41/2  "u(10)_Vr_derise"
  Sk_Calculation5/2(x_Matrix) -> Cϕx_Calculation5/1(x_Matrix), X_matrix3/1  "x_Matrix"
  Repeating Sequence Stair3/1 -> Ideal Switch3/1
  Mux43/1 -> u(k)_Calculation_1/1(u)
  E_0(理论值)5/1 -> Mux45/6  "u(6)_E_0"
  Mux42/1 -> Sk_Calculation5/1(u)
  δdelta(是一个大于最大扰动的值)5/1 -> Mux46/1  "δdelta"
  h(运算周期)7/1 -> Mux45/8  "u(5)_h"
  Repeating Sequence9/1 -> Mux44/1
  u(k)_Calculation_1/2(u_k_1) -> Transport Delay32/1
  h(运算周期)6/1 -> Mux45/7  "u(5)_h"
  Mux40/1 -> e2_Calculation6/1(u)
  Sine Wave11/1 -> Scope18/1  "u(10)_Vr_derise"
  Voltage Measurement4/1 -> Scope18/2, [v_o_7]
  MATLAB Function20/1(v_o) -> Mux41/1, Mux42/2, Mux40/3  "No_Consider_Disturbance"
  Sine Wave10/1 -> MATLAB Function24/1(u)  "u(10)_Vr_derise"
  Transport Delay31/1 -> Mux43/7  "u(7)_u_k-1"
  δ/ϕ_Calculation5/1(y) -> Mux43/4, δ/ϕ1/1  "u(4)_δ/ϕ"
  L(电感值)5/1 -> Mux45/1  "u(7)_L"
  [Q2_7] -> Mosfet19/1
  e1_Calculation6/1(Fact_e1) -> Mux40/7, Scope40/1, Mux42/3, Transport Delay35/1  "u(3)_e1(k)"
  (CΓ)'_Calculation5/4(D_Disturbance1_Matrix_k_2) -> Scope47/1
  Transport Delay34/1 -> (CΓ)'_Calculation5/3(D_k_1)
  Transport Delay33/1 -> Mux40/6
  Transport Delay32/1 -> 输出信号6/1
  [Q4_7] -> Mosfet18/1
  Vr_derise_d5/1 -> Mux40/2  "Vr_derise_d"
  MATLAB Function22/2(Q23) -> [Q2_7], [Q3_7]
  e2_Calculation6/4(Vo_RC) -> Scope36/2  "VO/RC"
  (CΓ)'_Calculation5/1(C_Gamma_Inv) -> C_Gamma_Inv1/1, Mux43/1  "u(1)_PhiC_Gamma_Inv"
  C(电容值)5/1 -> Mux40/4, Mux45/2  "u(8)_C"
  [v_o_4] -> To Workspace4/1, Scope48/1  "4"
  [v_o_7] -> To Workspace5/1, Scope48/2  "7"
  MATLAB Function26/1(flag) -> MATLAB Function25/1(flag)
  Repeating Sequence11/1 -> MATLAB Function25/2(compare_data)
  MATLAB Function25/1(Q14) -> Goto62/1, Goto61/1
  From79/1 -> MATLAB Function26/1(desert)
  MATLAB Function25/2(Q23) -> Goto63/1, Goto64/1
  Repeating Sequence Stair7/1 -> MATLAB Function27/1(u)  "u(10)_Vr_derise"
  From55/1 -> MATLAB Function28/1(u)
  MATLAB Function28/1(y) -> Mux37/15
  Repeating Sequence Stair9/1 -> MATLAB Function33/1(u)  "u(10)_Vr_derise"
  Mux47/1 -> e2_Calculation7/1(u)
  h(运算周期)8/1 -> Mux52/7  "u(5)_h"
  u(k)_Calculation_3/2(u_k_1) -> Transport Delay37/1
  Repeating Sequence13/1 -> Mux51/1
  h(运算周期)9/1 -> Mux52/8  "u(5)_h"
  E_0(理论值)6/1 -> Mux52/6  "u(6)_E_0"
  δdelta(是一个大于最大扰动的值)6/1 -> Mux53/1  "δdelta"
  Mux49/1 -> Sk_Calculation6/1(u)
  Repeating Sequence Stair8/1 -> Ideal Switch4/1
  Mux48/1 -> e1_Calculation7/1(u)
  Mux50/1 -> u(k)_Calculation_3/1(u)
  e2_Calculation7/3(iL_C) -> Scope52/1  "IL/C"
  Transport Delay36/1 -> Mux50/7  "u(7)_u_k-1"
  Voltage Measurement9/1 -> Scope50/2, [v_o_8]
  Mux51/1 -> MATLAB Function29/1(u)
  l(是一个大于零的数)6/1 -> Mux53/3  "l"
  Sk_Calculation6/1(Sk_Value) -> Scope53/1, Mux53/4, Sk3/1, Mux50/3  "conditional adpat SMC"
  不考虑扰动3/1 -> Mux50/6  "u(2)_alfa"
  e2_Calculation7/1(Fact_e2) -> Scope52/3, Scope51/1, Mux49/4, Transport Delay38/1  "(IL/C)-VO/RC"
  Cϕx_Calculation6/1(C_Phi_x) -> Cϕx3/1, Mux50/5  "u(5)_Cϕx"
  R_0(实际值)4/1 -> Mux52/3  "u(9)_R_0"
  u(k)_Calculation_3/1(u_k) -> Transport Delay36/1, Mux51/2  "u(k)"
  alfa(是一个0~1的数)6/1 -> Mux50/2  "u(2)_alfa"
  γgama(是一个0~1的数)6/1 -> Mux53/2  "γgama"
  MATLAB Function30/1(v_o) -> Mux48/1, Mux49/2, Mux47/3  "No_Consider_Disturbance"
  MATLAB Function33/1(y) -> Mux48/2  "u(10)_Vr_derise"
  (CΓ)'_Calculation6/2(Phi) -> Cϕx_Calculation6/2(Phi), Phi4/1  "Phi"
  R_0(理论值)6/1 -> Mux47/5, Mux52/4  "u(9)_R_0"
  [Q3_8] -> Mosfet32/1
  [u_k_8] -> MATLAB Function31/3(u)
  Current Measurement9/1 -> [i_l_8]
  MATLAB Function30/2(i_l) -> Mux49/1, Mux47/1  "Fact_i"
  Sk_Calculation6/2(x_Matrix) -> Cϕx_Calculation6/1(x_Matrix), X_matrix4/1  "x_Matrix"
  c_Matrix6/1 -> (CΓ)'_Calculation6/2(c), Sk_Calculation6/2(c), Cϕx_Calculation6/3(c_Matrix)  "c"
  Mux52/1 -> (CΓ)'_Calculation6/1(u)
  [i_l_8] -> MATLAB Function30/2(data)  "Fact_i"
  MATLAB Function32/1(flag) -> MATLAB Function31/1(flag)
  MATLAB Function31/1(Q14) -> [Q1_8], [Q4_8]
  Transport Delay40/1 -> Mux48/3
  Repeating Sequence12/1 -> MATLAB Function31/2(compare_data)
  (CΓ)'_Calculation6/3(D_Disturbance1_Matrix_k_1) -> Transport Delay39/1
  Sine Wave8/1 -> Scope50/1  "u(10)_Vr_derise"
  Mux53/1 -> δ/ϕ_Calculation6/1(u)
  e1_Calculation7/2(Last_e1) -> Mux47/8  "u(4)_e1(k-1)"
  [expect] -> MATLAB Function32/1(desert)
  (CΓ)'_Calculation6/1(C_Gamma_Inv) -> C_Gamma_Inv3/1, Mux50/1  "u(1)_PhiC_Gamma_Inv"
  [Q4_8] -> Mosfet26/1
  Transport Delay37/1 -> 输出信号7/1
  [v_o_8] -> MATLAB Function30/1(u)  "Fact_V"
  Vr_derise_d6/1 -> Mux47/2  "Vr_derise_d"
  MATLAB Function31/2(Q23) -> [Q2_8], [Q3_8]
  (CΓ)'_Calculation6/4(D_Disturbance1_Matrix_k_2) -> Scope57/1
  e2_Calculation7/4(Vo_RC) -> Scope52/2  "VO/RC"
  Transport Delay38/1 -> Mux47/6
  [Q1_8] -> Mosfet21/1
  MATLAB Function29/1(Output) -> Scope55/1, [u_k_8]  "gate"
  e1_Calculation7/1(Fact_e1) -> Mux47/7, Scope54/1, Mux49/3, Transport Delay40/1  "u(3)_e1(k)"
  Transport Delay39/1 -> (CΓ)'_Calculation6/3(D_k_1)
  E(实际的值)6/1 -> Mux52/5
  [Q2_8] -> Mosfet31/1
  C(电容值)6/1 -> Mux47/4, Mux52/2  "u(8)_C"
  δ/ϕ_Calculation6/1(y) -> Mux50/4, δ/ϕ3/1  "u(4)_δ/ϕ"
  L(电感值)6/1 -> Mux52/1  "u(7)_L"
  u(k)_Calculation_3/6(Disturbance) -> Scope56/1
  [v_o_8] -> Scope48/3  "最坏的"
  [v_o_6] -> To Workspace6/1, Scope48/4  "最好的"
  [Sk_1] -> To Workspace7/1, Scope59/1  "1"
  [Sk_2] -> To Workspace8/1, Scope59/2  "2"
  Sine Wave4/1 -> Scope61/1  "u(10)_Vr_derise"
  connections:
  DC Voltage Source2/RConn1 -- Mosfet3/LConn1 -- Mosfet5/LConn1
  Mosfet3/RConn1 -- Series RLC Branch12/LConn1 -- Mosfet2/LConn1
  Voltage Measurement6/LConn2 -- Ideal Switch/LConn1 -- Series RLC Branch14/RConn1 -- Series RLC Branch13/RConn1 -- Mosfet5/RConn1 -- Mosfet4/LConn1
  DC Voltage Source2/LConn1 -- Mosfet4/RConn1 -- Mosfet2/RConn1
  Series RLC Branch14/LConn1 -- Series RLC Branch10/LConn1 -- Voltage Measurement6/LConn1 -- Current Measurement5/RConn1 -- Series RLC Branch13/LConn1
  Current Measurement5/LConn1 -- Series RLC Branch12/RConn1
  Series RLC Branch3/RConn1 -- Voltage Measurement1/LConn2 -- Current Measurement1/LConn1
  Mosfet1/RConn1 -- DC Voltage Source1/LConn1 -- Mosfet7/RConn1
  Current Measurement1/RConn1 -- Mosfet8/RConn1 -- Mosfet7/LConn1 -- Series RLC Branch2/RConn1
  Mosfet8/LConn1 -- DC Voltage Source1/RConn1 -- Mosfet6/LConn1
  Series RLC Branch2/LConn1 -- Series RLC Branch3/LConn1 -- Voltage Measurement1/LConn1 -- Current Measurement2/RConn1
  Mosfet1/LConn1 -- Mosfet6/RConn1 -- Series RLC Branch1/LConn1
  Current Measurement2/LConn1 -- Series RLC Branch1/RConn1
  Series RLC Branch5/LConn1 -- Current Measurement6/RConn1 -- Series RLC Branch6/LConn1 -- Voltage Measurement2/LConn1
  Mosfet9/RConn1 -- DC Voltage Source3/LConn1 -- Mosfet11/RConn1
  Mosfet9/LConn1 -- Mosfet10/RConn1 -- Series RLC Branch4/LConn1
  Series RLC Branch6/RConn1 -- Voltage Measurement2/LConn2 -- Current Measurement3/LConn1
  Mosfet12/LConn1 -- DC Voltage Source3/RConn1 -- Mosfet10/LConn1
  Current Measurement3/RConn1 -- Series RLC Branch5/RConn1 -- Mosfet12/RConn1 -- Mosfet11/LConn1
  Current Measurement6/LConn1 -- Series RLC Branch4/RConn1
  Mosfet13/LConn1 -- Mosfet15/LConn1 -- DC Voltage Source4/RConn1
  Voltage Measurement3/LConn2 -- Ideal Switch1/LConn1 -- Series RLC Branch9/RConn1 -- Series RLC Branch8/RConn1 -- Mosfet15/RConn1 -- Mosfet14/LConn1
  Series RLC Branch7/LConn1 -- Mosfet16/LConn1 -- Mosfet13/RConn1
  Voltage Measurement3/LConn1 -- Series RLC Branch11/LConn1 -- Series RLC Branch9/LConn1 -- Series RLC Branch8/LConn1 -- Current Measurement8/RConn1
  Mosfet14/RConn1 -- Mosfet16/RConn1 -- DC Voltage Source4/LConn1
  Current Measurement8/LConn1 -- Series RLC Branch7/RConn1
  Voltage Measurement7/LConn1 -- Series RLC Branch22/LConn1 -- Current Measurement13/RConn1 -- Series RLC Branch21/LConn1
  Mosfet23/LConn1 -- Mosfet24/RConn1 -- Current Measurement12/RConn1 -- Series RLC Branch21/RConn1
  Mosfet23/RConn1 -- Mosfet25/RConn1 -- DC Voltage Source7/LConn1
  Series RLC Branch20/LConn1 -- Mosfet25/LConn1 -- Mosfet22/RConn1
  Current Measurement12/LConn1 -- Series RLC Branch22/RConn1 -- Voltage Measurement7/LConn2
  Mosfet22/LConn1 -- Mosfet24/LConn1 -- DC Voltage Source7/RConn1
  Current Measurement13/LConn1 -- Series RLC Branch20/RConn1
  Series RLC Branch10/RConn1 -- Ideal Switch/RConn1
  Series RLC Branch11/RConn1 -- Ideal Switch1/RConn1
  Mosfet30/RConn1 -- Mosfet29/LConn1 -- Diode2/LConn1 -- Voltage Measurement8/LConn2 -- Series RLC Branch25/RConn1 -- Series RLC Branch24/RConn1
  Voltage Measurement8/LConn1 -- Series RLC Branch25/LConn1 -- Current Measurement7/RConn1 -- Series RLC Branch24/LConn1 -- Series RLC Branch19/LConn1
  Current Measurement7/LConn1 -- Series RLC Branch23/RConn1
  Series RLC Branch19/RConn1 -- Ideal Switch2/RConn1
  Mosfet27/RConn1 -- DC Voltage Source9/LConn1 -- Voltage Measurement5/LConn2 -- Mosfet29/RConn1
  Mosfet30/LConn1 -- Voltage Measurement5/LConn1 -- DC Voltage Source9/RConn1 -- Mosfet28/LConn1
  Mosfet28/RConn1 -- Mosfet27/LConn1 -- Diode2/RConn1 -- Series RLC Branch23/LConn1
  Current Measurement4/RConn1 -- Series RLC Branch17/LConn1 -- Voltage Measurement4/LConn1 -- Series RLC Branch15/LConn1 -- Series RLC Branch18/LConn1
  Series RLC Branch18/RConn1 -- Voltage Measurement4/LConn2 -- Ideal Switch3/LConn1 -- Mosfet19/RConn1 -- Mosfet18/LConn1 -- Series RLC Branch17/RConn1
  Mosfet17/RConn1 -- Series RLC Branch16/LConn1 -- Mosfet20/LConn1
  DC Voltage Source5/RConn1 -- Mosfet17/LConn1 -- Mosfet19/LConn1
  DC Voltage Source5/LConn1 -- Mosfet18/RConn1 -- Mosfet20/RConn1
  Series RLC Branch15/RConn1 -- Ideal Switch3/RConn1
  Current Measurement4/LConn1 -- Series RLC Branch16/RConn1
  DC Voltage Source6/LConn1 -- Mosfet26/RConn1 -- Mosfet32/RConn1
  Series RLC Branch29/RConn1 -- Mosfet31/RConn1 -- Mosfet26/LConn1 -- Series RLC Branch28/RConn1 -- Voltage Measurement9/LConn2 -- Ideal Switch4/LConn1
  DC Voltage Source6/RConn1 -- Mosfet21/LConn1 -- Mosfet31/LConn1
  Mosfet21/RConn1 -- Series RLC Branch27/LConn1 -- Mosfet32/LConn1
  Series RLC Branch29/LConn1 -- Voltage Measurement9/LConn1 -- Series RLC Branch26/LConn1 -- Series RLC Branch28/LConn1 -- Current Measurement9/RConn1
  Current Measurement9/LConn1 -- Series RLC Branch27/RConn1
  Series RLC Branch26/RConn1 -- Ideal Switch4/RConn1
